simulink model "c_ss_cl"  (Simulink 5.0)
settings: Solver=ode45  StartTime=t_init  StopTime=t_final  RelTol=1e-3
values from neighbouring files (symbols this model uses):
  b = a(length(a):-1:1)    [flip.m]    (also in indep.m = [-c 1]; t1calc.m = move(b,find(sel),Srows))
  c = makezero(c,gap)    [indep.m]
undefined symbols (not defined in the file or in its folder): a, C, D, d, gamma, N, N_var, Rc, Sc, st, Tc, Ts, xInitial
settings Model: Creator=kannan  LastModifiedBy=kannan  ExtModeAutoUpdateStatusClock=off

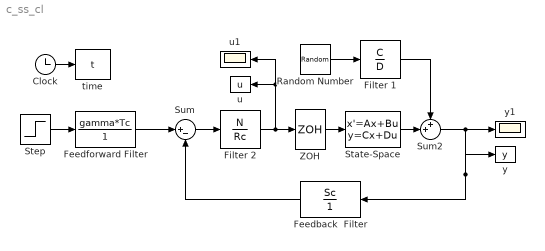
== system c_ss_cl ==
  " Filter 2" : DiscreteFilter  Numerator=N  Denominator=Rc  SampleTime=Ts
  Clock : Clock
      settings: Decimation=10
  Feedback  Filter : DiscreteFilter  Orientation=left  Numerator=Sc  Denominator=1  SampleTime=Ts
  Feedforward Filter : DiscreteFilter  Numerator=gamma*Tc  Denominator=1  SampleTime=Ts
  Filter 1 : DiscreteFilter  Numerator=C  Denominator=D  SampleTime=Ts
  Random Number : RandomNumber  Variance=N_var  SampleTime=Ts
  State-Space : StateSpace  A=a  B=b  C=c  D=d  X0=xInitial
  Step : Step  Time=0  After=st  SampleTime=Ts
  Sum : Sum  Inputs=|+-  SaturateOnIntegerOverflow=on
  Sum2 : Sum  Inputs=++|  SaturateOnIntegerOverflow=on
  ZOH : ZeroOrderHold  SampleTime=Ts
  time : ToWorkspace  VariableName=t  SampleTime=Ts  SaveFormat=Array
  u : ToWorkspace  VariableName=u  SampleTime=Ts  SaveFormat=Array
  u1 : Scope
      settings: YMin=-6e+164  YMax=1.02293e+149
  y : ToWorkspace  VariableName=y  SampleTime=Ts  SaveFormat=Array
  y1 : Scope
      settings: YMin=-6e+164  YMax=1.02293e+149
  wires:
  Feedforward Filter/1 -> Sum/1
  Feedback  Filter/1 -> Sum/2
  Clock/1 -> time/1
  State-Space/1 -> Sum2/2
  Filter 1/1 -> Sum2/1
  Random Number/1 -> Filter 1/1
  Sum2/1 -> y1/1, Feedback  Filter/1, y/1
  Sum/1 -> " Filter 2"/1
  " Filter 2"/1 -> u1/1, u/1, ZOH/1
  ZOH/1 -> State-Space/1
  Step/1 -> Feedforward Filter/1
